simulink model "forward_VAE"  (R2021b)
settings: Solver=FixedStepDiscrete  StartTime=0.0  StopTime=10.0  RelTol=1e-3
PreLoadFcn:
  | CWL=24;
  | CFL=16;
  | CWL_W2=32;
  | CFL_W2=24;
  | CWL_W3=32;
  | CFL_W3=24;
InitFcn:
  | CWL=24;
  | CFL=16;
  | CWL_W2=32;
  | CFL_W2=24;
  | CWL_W3=32;
  | CFL_W3=24;
settings Model: Creator=Kuro  LastModifiedBy=Kuro
settings SolverCC: AlgebraicLoopSolver=TrustRegion
settings OptimizationCC: BlockReduction=off  ConditionallyExecuteInputs=off  DefaultParameterBehavior=Inlined
settings DebuggingCC: AlgebraicLoopMsg=error  SFMachineParentedDataDiag=warning
settings HardwareCC: ProdBitPerPointer=32  ProdBitPerSizeT=32  ProdBitPerPtrDiffT=32  ProdLargestAtomicFloat=None  ProdIntDivRoundTo=Undefined  ProdEndianess=Unspecified  ProdWordSize=32  ProdHWDeviceType=ASIC/FPGA->ASIC/FPGA  TargetBitPerPointer=64  TargetBitPerSizeT=64  TargetBitPerPtrDiffT=64  TargetLongLongMode=on  TargetIntDivRoundTo=Zero  TargetEndianess=LittleEndian  TargetWordSize=64  TargetHWDeviceType=Custom Processor->MATLAB Host Computer  ProdEqTarget=off

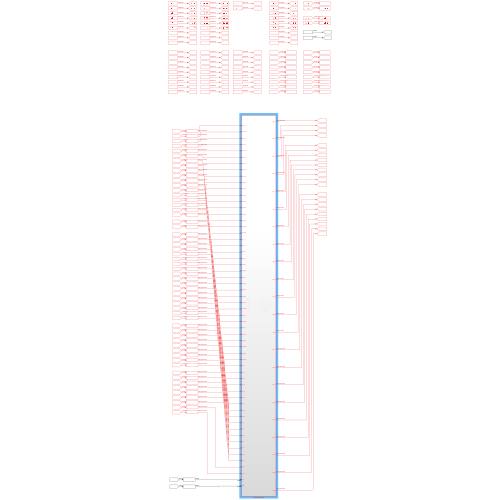
[thumbnail: Simulink's stored preview of the top-level diagram]
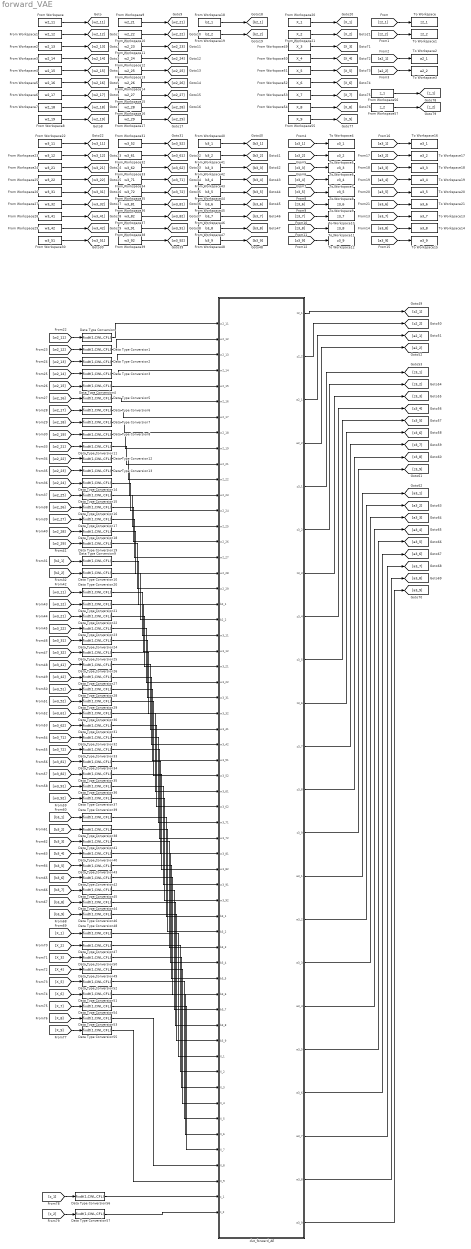
== system forward_VAE ==
  Data Type Conversion{,1..57} (58 alike) : DataTypeConversion  OutDataTypeStr=fixdt(1,CWL,CFL)  SaturateOnIntegerOverflow=on
  From Workspace : FromWorkspace  VariableName=w2_11  SampleTime=1
  From Workspace1 : FromWorkspace  VariableName=w2_12  SampleTime=1
  From Workspace10 : FromWorkspace  VariableName=w2_22  SampleTime=1
  From Workspace11 : FromWorkspace  VariableName=w2_23  SampleTime=1
  From Workspace12 : FromWorkspace  VariableName=w2_24  SampleTime=1
  From Workspace13 : FromWorkspace  VariableName=w2_25  SampleTime=1
  From Workspace14 : FromWorkspace  VariableName=w2_26  SampleTime=1
  From Workspace15 : FromWorkspace  VariableName=w2_27  SampleTime=1
  From Workspace16 : FromWorkspace  VariableName=w2_28  SampleTime=1
  From Workspace17 : FromWorkspace  VariableName=w2_29  SampleTime=1
  From Workspace18 : FromWorkspace  VariableName=b2_1  SampleTime=1
  From Workspace19 : FromWorkspace  VariableName=b2_2  SampleTime=1
  From Workspace2 : FromWorkspace  VariableName=w2_13  SampleTime=1
  From Workspace20 : FromWorkspace  VariableName=X_1  SampleTime=1
  From Workspace21 : FromWorkspace  VariableName=X_2  SampleTime=1
  From Workspace22 : FromWorkspace  VariableName=w3_11  SampleTime=1
  From Workspace23 : FromWorkspace  VariableName=w3_12  SampleTime=1
  From Workspace24 : FromWorkspace  VariableName=w3_21  SampleTime=1
  From Workspace25 : FromWorkspace  VariableName=w3_22  SampleTime=1
  From Workspace26 : FromWorkspace  VariableName=w3_31  SampleTime=1
  From Workspace27 : FromWorkspace  VariableName=w3_32  SampleTime=1
  From Workspace28 : FromWorkspace  VariableName=w3_41  SampleTime=1
  From Workspace29 : FromWorkspace  VariableName=w3_42  SampleTime=1
  From Workspace3 : FromWorkspace  VariableName=w2_14  SampleTime=1
  From Workspace30 : FromWorkspace  VariableName=w3_51  SampleTime=1
  From Workspace31 : FromWorkspace  VariableName=w3_52  SampleTime=1
  From Workspace32 : FromWorkspace  VariableName=w3_61  SampleTime=1
  From Workspace33 : FromWorkspace  VariableName=w3_62  SampleTime=1
  From Workspace34 : FromWorkspace  VariableName=w3_71  SampleTime=1
  From Workspace35 : FromWorkspace  VariableName=w3_72  SampleTime=1
  From Workspace36 : FromWorkspace  VariableName=w3_81  SampleTime=1
  From Workspace37 : FromWorkspace  VariableName=w3_82  SampleTime=1
  From Workspace38 : FromWorkspace  VariableName=w3_91  SampleTime=1
  From Workspace39 : FromWorkspace  VariableName=w3_92  SampleTime=1
  From Workspace4 : FromWorkspace  VariableName=w2_15  SampleTime=1
  From Workspace40 : FromWorkspace  VariableName=b3_1  SampleTime=1
  From Workspace41 : FromWorkspace  VariableName=b3_2  SampleTime=1
  From Workspace42 : FromWorkspace  VariableName=b3_3  SampleTime=1
  From Workspace43 : FromWorkspace  VariableName=b3_4  SampleTime=1
  From Workspace44 : FromWorkspace  VariableName=b3_5  SampleTime=1
  From Workspace45 : FromWorkspace  VariableName=b3_6  SampleTime=1
  From Workspace46 : FromWorkspace  VariableName=b3_7  SampleTime=1
  From Workspace47 : FromWorkspace  VariableName=b3_8  SampleTime=1
  From Workspace48 : FromWorkspace  VariableName=b3_9  SampleTime=1
  From Workspace49 : FromWorkspace  VariableName=X_3  SampleTime=1
  From Workspace5 : FromWorkspace  VariableName=w2_16  SampleTime=1
  From Workspace50 : FromWorkspace  VariableName=X_4  SampleTime=1
  From Workspace51 : FromWorkspace  VariableName=X_5  SampleTime=1
  From Workspace52 : FromWorkspace  VariableName=X_6  SampleTime=1
  From Workspace53 : FromWorkspace  VariableName=X_7  SampleTime=1
  From Workspace54 : FromWorkspace  VariableName=X_8  SampleTime=1
  From Workspace55 : FromWorkspace  VariableName=X_9  SampleTime=1
  From Workspace56 : FromWorkspace  VariableName=z_1  SampleTime=1
  From Workspace57 : FromWorkspace  VariableName=z_2  SampleTime=1
  From Workspace6 : FromWorkspace  VariableName=w2_17  SampleTime=1
  From Workspace7 : FromWorkspace  VariableName=w2_18  SampleTime=1
  From Workspace8 : FromWorkspace  VariableName=w2_19  SampleTime=1
  From Workspace9 : FromWorkspace  VariableName=w2_21  SampleTime=1
  To Workspace : ToWorkspace  VariableName=z2_1  SaveFormat=Timeseries  SampleTime=-1
  To Workspace1 : ToWorkspace  VariableName=z2_2  SaveFormat=Timeseries  SampleTime=-1
  To Workspace10 : ToWorkspace  VariableName=z3_7  SaveFormat=Timeseries  SampleTime=-1
  To Workspace11 : ToWorkspace  VariableName=z3_8  SaveFormat=Timeseries  SampleTime=-1
  To Workspace12 : ToWorkspace  VariableName=z3_9  SaveFormat=Timeseries  SampleTime=-1
  To Workspace13 : ToWorkspace  VariableName=a3_7  SaveFormat=Timeseries  SampleTime=-1
  To Workspace14 : ToWorkspace  VariableName=a3_8  SaveFormat=Timeseries  SampleTime=-1
  To Workspace15 : ToWorkspace  VariableName=a3_9  SaveFormat=Timeseries  SampleTime=-1
  To Workspace16 : ToWorkspace  VariableName=a3_1  SaveFormat=Timeseries  SampleTime=-1
  To Workspace17 : ToWorkspace  VariableName=a3_2  SaveFormat=Timeseries  SampleTime=-1
  To Workspace18 : ToWorkspace  VariableName=a3_3  SaveFormat=Timeseries  SampleTime=-1
  To Workspace19 : ToWorkspace  VariableName=a3_4  SaveFormat=Timeseries  SampleTime=-1
  To Workspace2 : ToWorkspace  VariableName=a2_1  SaveFormat=Timeseries  SampleTime=-1
  To Workspace20 : ToWorkspace  VariableName=a3_5  SaveFormat=Timeseries  SampleTime=-1
  To Workspace21 : ToWorkspace  VariableName=a3_6  SaveFormat=Timeseries  SampleTime=-1
  To Workspace3 : ToWorkspace  VariableName=a2_2  SaveFormat=Timeseries  SampleTime=-1
  To Workspace4 : ToWorkspace  VariableName=z3_1  SaveFormat=Timeseries  SampleTime=-1
  To Workspace5 : ToWorkspace  VariableName=z3_2  SaveFormat=Timeseries  SampleTime=-1
  To Workspace6 : ToWorkspace  VariableName=z3_3  SaveFormat=Timeseries  SampleTime=-1
  To Workspace7 : ToWorkspace  VariableName=z3_4  SaveFormat=Timeseries  SampleTime=-1
  To Workspace8 : ToWorkspace  VariableName=z3_5  SaveFormat=Timeseries  SampleTime=-1
  To Workspace9 : ToWorkspace  VariableName=z3_6  SaveFormat=Timeseries  SampleTime=-1
  dut_forward_AE : Subsystem  TreatAsAtomicUnit=on
  wires:
  From Workspace/1 -> [w2_11]
  From Workspace1/1 -> [w2_12]
  From Workspace3/1 -> [w2_14]
  From Workspace2/1 -> [w2_13]
  From Workspace6/1 -> [w2_17]
  From Workspace5/1 -> [w2_16]
  From Workspace4/1 -> [w2_15]
  From Workspace7/1 -> [w2_18]
  From Workspace8/1 -> [w2_19]
  From Workspace17/1 -> [w2_29]
  From Workspace16/1 -> [w2_28]
  From Workspace13/1 -> [w2_25]
  From Workspace14/1 -> [w2_26]
  From Workspace15/1 -> [w2_27]
  From Workspace11/1 -> [w2_23]
  From Workspace12/1 -> [w2_24]
  From Workspace10/1 -> [w2_22]
  From Workspace9/1 -> [w2_21]
  From Workspace18/1 -> [b2_1]
  From Workspace19/1 -> [b2_2]
  From Workspace30/1 -> [w3_51]
  From Workspace29/1 -> [w3_42]
  From Workspace26/1 -> [w3_31]
  From Workspace27/1 -> [w3_32]
  From Workspace28/1 -> [w3_41]
  From Workspace24/1 -> [w3_21]
  From Workspace25/1 -> [w3_22]
  From Workspace23/1 -> [w3_12]
  From Workspace22/1 -> [w3_11]
  From Workspace31/1 -> [w3_52]
  From Workspace33/1 -> [w3_62]
  From Workspace32/1 -> [w3_61]
  From Workspace36/1 -> [w3_81]
  From Workspace35/1 -> [w3_72]
  From Workspace34/1 -> [w3_71]
  From Workspace37/1 -> [w3_82]
  From Workspace38/1 -> [w3_91]
  From Workspace39/1 -> [w3_92]
  From Workspace40/1 -> [b3_1]
  From Workspace41/1 -> [b3_2]
  From Workspace43/1 -> [b3_4]
  From Workspace42/1 -> [b3_3]
  From Workspace46/1 -> [b3_7]
  From Workspace47/1 -> [b3_8]
  From Workspace45/1 -> [b3_6]
  From Workspace44/1 -> [b3_5]
  From Workspace48/1 -> [b3_9]
  [z2_1] -> To Workspace/1
  [z2_2] -> To Workspace1/1
  [a2_2] -> To Workspace3/1
  [a2_1] -> To Workspace2/1
  [z3_2] -> To Workspace5/1
  [z3_1] -> To Workspace4/1
  [z3_3] -> To Workspace6/1
  [z3_4] -> To Workspace7/1
  [z3_8] -> To Workspace11/1
  [z3_7] -> To Workspace10/1
  [z3_5] -> To Workspace8/1
  [z3_6] -> To Workspace9/1
  [z3_9] -> To Workspace12/1
  [a3_9] -> To Workspace15/1
  [a3_6] -> To Workspace21/1
  [a3_5] -> To Workspace20/1
  [a3_7] -> To Workspace13/1
  [a3_8] -> To Workspace14/1
  [a3_4] -> To Workspace19/1
  [a3_3] -> To Workspace18/1
  [a3_1] -> To Workspace16/1
  [a3_2] -> To Workspace17/1
  [w2_11] -> Data Type Conversion/1
  [w2_12] -> Data Type Conversion1/1
  [w2_14] -> Data Type Conversion3/1
  [w2_13] -> Data Type Conversion2/1
  [w2_17] -> Data Type Conversion6/1
  [w2_18] -> Data Type Conversion7/1
  [w2_16] -> Data Type Conversion5/1
  [w2_15] -> Data Type Conversion4/1
  [w2_19] -> Data Type Conversion8/1
  [b2_1] -> Data Type Conversion9/1
  [w2_29] -> Data Type Conversion19/1
  [w2_25] -> Data Type Conversion15/1
  [w2_26] -> Data Type Conversion16/1
  [w2_28] -> Data Type Conversion18/1
  [w2_27] -> Data Type Conversion17/1
  [w2_23] -> Data Type Conversion13/1
  [w2_24] -> Data Type Conversion14/1
  [w2_22] -> Data Type Conversion12/1
  [w2_21] -> Data Type Conversion11/1
  [b2_2] -> Data Type Conversion10/1
  [w3_12] -> Data Type Conversion21/1
  [w3_11] -> Data Type Conversion20/1
  [w3_21] -> Data Type Conversion22/1
  [w3_22] -> Data Type Conversion23/1
  [w3_42] -> Data Type Conversion27/1
  [w3_41] -> Data Type Conversion26/1
  [w3_31] -> Data Type Conversion24/1
  [w3_32] -> Data Type Conversion25/1
  [w3_72] -> Data Type Conversion33/1
  [w3_71] -> Data Type Conversion32/1
  [w3_81] -> Data Type Conversion34/1
  [w3_62] -> Data Type Conversion31/1
  [w3_61] -> Data Type Conversion30/1
  [w3_51] -> Data Type Conversion28/1
  [w3_52] -> Data Type Conversion29/1
  [w3_82] -> Data Type Conversion35/1
  [w3_92] -> Data Type Conversion37/1
  [w3_91] -> Data Type Conversion36/1
  [b3_2] -> Data Type Conversion38/1
  [b3_1] -> Data Type Conversion39/1
  [b3_3] -> Data Type Conversion41/1
  [b3_4] -> Data Type Conversion40/1
  [b3_8] -> Data Type Conversion44/1
  [b3_7] -> Data Type Conversion45/1
  [b3_5] -> Data Type Conversion43/1
  [b3_6] -> Data Type Conversion42/1
  [b3_9] -> Data Type Conversion46/1
  [X_1] -> Data Type Conversion48/1
  [X_2] -> Data Type Conversion47/1
  From Workspace55/1 -> [X_9]
  From Workspace51/1 -> [X_5]
  From Workspace52/1 -> [X_6]
  From Workspace54/1 -> [X_8]
  From Workspace53/1 -> [X_7]
  From Workspace49/1 -> [X_3]
  From Workspace50/1 -> [X_4]
  From Workspace21/1 -> [X_2]
  From Workspace20/1 -> [X_1]
  [X_4] -> Data Type Conversion49/1
  [X_3] -> Data Type Conversion50/1
  [X_7] -> Data Type Conversion54/1
  [X_8] -> Data Type Conversion53/1
  [X_6] -> Data Type Conversion51/1
  [X_5] -> Data Type Conversion52/1
  [X_9] -> Data Type Conversion55/1
  Data Type Conversion/1 -> dut_forward_AE/1(w2_11)
  Data Type Conversion1/1 -> dut_forward_AE/2(w2_12)
  Data Type Conversion2/1 -> dut_forward_AE/3(w2_13)
  Data Type Conversion3/1 -> dut_forward_AE/4(w2_14)
  Data Type Conversion4/1 -> dut_forward_AE/5(w2_15)
  Data Type Conversion5/1 -> dut_forward_AE/6(w2_16)
  Data Type Conversion6/1 -> dut_forward_AE/7(w2_17)
  Data Type Conversion7/1 -> dut_forward_AE/8(w2_18)
  Data Type Conversion8/1 -> dut_forward_AE/9(w2_19)
  Data Type Conversion11/1 -> dut_forward_AE/10(w2_21)
  Data Type Conversion12/1 -> dut_forward_AE/11(w2_22)
  Data Type Conversion13/1 -> dut_forward_AE/12(w2_23)
  Data Type Conversion14/1 -> dut_forward_AE/13(w2_24)
  Data Type Conversion15/1 -> dut_forward_AE/14(w2_25)
  Data Type Conversion16/1 -> dut_forward_AE/15(w2_26)
  Data Type Conversion17/1 -> dut_forward_AE/16(w2_27)
  Data Type Conversion18/1 -> dut_forward_AE/17(w2_28)
  Data Type Conversion19/1 -> dut_forward_AE/18(w2_29)
  Data Type Conversion9/1 -> dut_forward_AE/19(b2_1)
  Data Type Conversion10/1 -> dut_forward_AE/20(b2_2)
  Data Type Conversion20/1 -> dut_forward_AE/21(w3_11)
  Data Type Conversion21/1 -> dut_forward_AE/22(w3_12)
  Data Type Conversion22/1 -> dut_forward_AE/23(w3_21)
  Data Type Conversion23/1 -> dut_forward_AE/24(w3_22)
  Data Type Conversion24/1 -> dut_forward_AE/25(w3_31)
  Data Type Conversion25/1 -> dut_forward_AE/26(w3_32)
  Data Type Conversion26/1 -> dut_forward_AE/27(w3_41)
  Data Type Conversion27/1 -> dut_forward_AE/28(w3_42)
  Data Type Conversion28/1 -> dut_forward_AE/29(w3_51)
  Data Type Conversion29/1 -> dut_forward_AE/30(w3_52)
  Data Type Conversion30/1 -> dut_forward_AE/31(w3_61)
  Data Type Conversion31/1 -> dut_forward_AE/32(w3_62)
  Data Type Conversion32/1 -> dut_forward_AE/33(w3_71)
  Data Type Conversion33/1 -> dut_forward_AE/34(w3_72)
  Data Type Conversion34/1 -> dut_forward_AE/35(w3_81)
  Data Type Conversion35/1 -> dut_forward_AE/36(w3_82)
  Data Type Conversion36/1 -> dut_forward_AE/37(w3_91)
  Data Type Conversion37/1 -> dut_forward_AE/38(w3_92)
  Data Type Conversion39/1 -> dut_forward_AE/39(b3_1)
  Data Type Conversion38/1 -> dut_forward_AE/40(b3_2)
  Data Type Conversion41/1 -> dut_forward_AE/41(b3_3)
  Data Type Conversion40/1 -> dut_forward_AE/42(b3_4)
  Data Type Conversion43/1 -> dut_forward_AE/43(b3_5)
  Data Type Conversion42/1 -> dut_forward_AE/44(b3_6)
  Data Type Conversion45/1 -> dut_forward_AE/45(b3_7)
  Data Type Conversion44/1 -> dut_forward_AE/46(b3_8)
  Data Type Conversion46/1 -> dut_forward_AE/47(b3_9)
  Data Type Conversion48/1 -> dut_forward_AE/48(X_1)
  Data Type Conversion47/1 -> dut_forward_AE/49(X_2)
  Data Type Conversion50/1 -> dut_forward_AE/50(X_3)
  Data Type Conversion49/1 -> dut_forward_AE/51(X_4)
  Data Type Conversion52/1 -> dut_forward_AE/52(X_5)
  Data Type Conversion51/1 -> dut_forward_AE/53(X_6)
  Data Type Conversion54/1 -> dut_forward_AE/54(X_7)
  Data Type Conversion53/1 -> dut_forward_AE/55(X_8)
  Data Type Conversion55/1 -> dut_forward_AE/56(X_9)
  dut_forward_AE/1(z2_1) -> [z2_1]
  dut_forward_AE/2(z2_2) -> [z2_2]
  dut_forward_AE/3(a2_1) -> [a2_1]
  dut_forward_AE/4(a2_2) -> [a2_2]
  dut_forward_AE/5(z3_1) -> [z3_1]
  dut_forward_AE/6(z3_2) -> [z3_2]
  dut_forward_AE/7(z3_3) -> [z3_3]
  dut_forward_AE/8(z3_4) -> [z3_4]
  dut_forward_AE/9(z3_5) -> [z3_5]
  dut_forward_AE/10(z3_6) -> [z3_6]
  dut_forward_AE/11(z3_7) -> [z3_7]
  dut_forward_AE/12(z3_8) -> [z3_8]
  dut_forward_AE/13(z3_9) -> [z3_9]
  dut_forward_AE/14(a3_1) -> [a3_1]
  dut_forward_AE/15(a3_2) -> [a3_2]
  dut_forward_AE/16(a3_3) -> [a3_3]
  dut_forward_AE/17(a3_4) -> [a3_4]
  dut_forward_AE/18(a3_5) -> [a3_5]
  dut_forward_AE/19(a3_6) -> [a3_6]
  dut_forward_AE/20(a3_7) -> [a3_7]
  dut_forward_AE/21(a3_8) -> [a3_8]
  dut_forward_AE/22(a3_9) -> [a3_9]
  From Workspace56/1 -> [z_1]
  From Workspace57/1 -> [z_2]
  [z_1] -> Data Type Conversion56/1
  [z_2] -> Data Type Conversion57/1
  Data Type Conversion56/1 -> dut_forward_AE/57(z_1)
  Data Type Conversion57/1 -> dut_forward_AE/58(z_2)

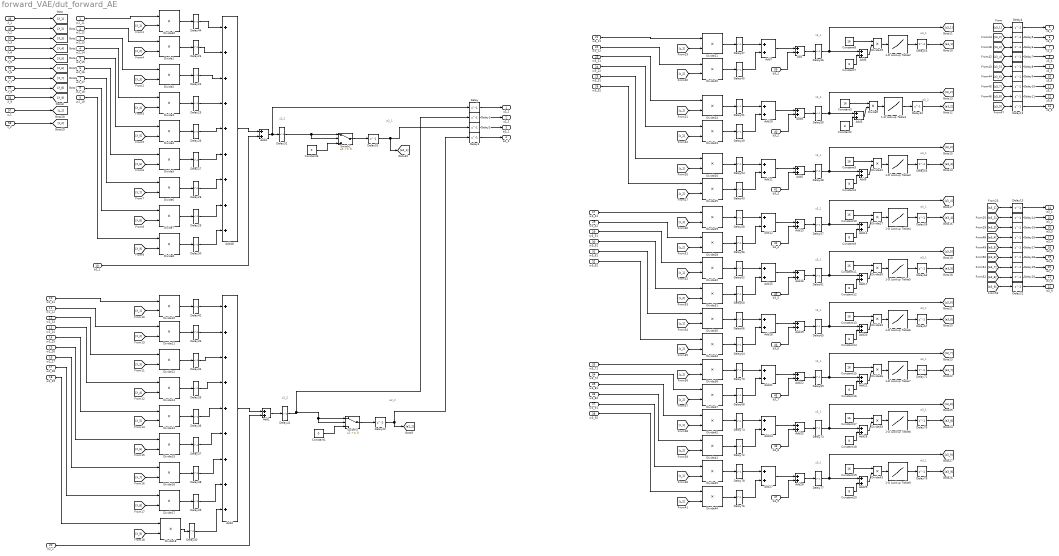
== system forward_VAE/dut_forward_AE ==
  note: a2_1
  note: z2_1
  note: a2_2
  note: z2_2
  note: z3_1
  note: a3_1
  note: z3_2
  note: a3_2
  note: z3_1
  note: a3_1
  note: z3_1
  note: a3_1
  note: z3_1
  note: a3_1
  note: z3_1
  note: a3_1
  note: z3_1
  note: a3_1
  note: z3_1
  note: a3_1
  note: z3_1
  note: a3_1
  w2_11 : Inport
  w2_12 : Inport  Port=2
  w2_13 : Inport  Port=3
  w2_14 : Inport  Port=4
  w2_15 : Inport  Port=5
  w2_16 : Inport  Port=6
  w2_17 : Inport  Port=7
  w2_18 : Inport  Port=8
  w2_19 : Inport  Port=9
  w2_21 : Inport  Port=10
  w2_22 : Inport  Port=11
  w2_23 : Inport  Port=12
  w2_24 : Inport  Port=13
  w2_25 : Inport  Port=14
  w2_26 : Inport  Port=15
  w2_27 : Inport  Port=16
  w2_28 : Inport  Port=17
  w2_29 : Inport  Port=18
  b2_1 : Inport  Port=19
  b2_2 : Inport  Port=20
  w3_11 : Inport  Port=21
  w3_12 : Inport  Port=22
  w3_21 : Inport  Port=23
  w3_22 : Inport  Port=24
  w3_31 : Inport  Port=25
  w3_32 : Inport  Port=26
  w3_41 : Inport  Port=27
  w3_42 : Inport  Port=28
  w3_51 : Inport  Port=29
  w3_52 : Inport  Port=30
  w3_61 : Inport  Port=31
  w3_62 : Inport  Port=32
  w3_71 : Inport  Port=33
  w3_72 : Inport  Port=34
  w3_81 : Inport  Port=35
  w3_82 : Inport  Port=36
  w3_91 : Inport  Port=37
  w3_92 : Inport  Port=38
  b3_1 : Inport  Port=39
  b3_2 : Inport  Port=40
  b3_3 : Inport  Port=41
  b3_4 : Inport  Port=42
  b3_5 : Inport  Port=43
  b3_6 : Inport  Port=44
  b3_7 : Inport  Port=45
  b3_8 : Inport  Port=46
  b3_9 : Inport  Port=47
  X_1 : Inport  Port=48
  X_2 : Inport  Port=49
  X_3 : Inport  Port=50
  X_4 : Inport  Port=51
  X_5 : Inport  Port=52
  X_6 : Inport  Port=53
  X_7 : Inport  Port=54
  X_8 : Inport  Port=55
  X_9 : Inport  Port=56
  z_1 : Inport  Port=57
  z_2 : Inport  Port=58
  1-D Lookup Table{1..9} (9 alike) : Lookup_n-D  NumberOfTableDimensions=1  LookupTableObject=''  BreakpointsForDimension1=[0:255]  BreakpointsForDimension1FirstPoint=10  BreakpointsForDimension2FirstPoint=10  BreakpointsForDimension1Spacing=12  BreakpointsForDimension2Spacing=12  IndexSearchMethod=Evenly spaced points  Table=1./(1+exp(-1*[-8:2^(-4):8-2^(-4)]))  InterpMethod=Flat  DiagnosticForOutOfRangeInput=Error  OutDataTypeStr=fixdt(1,CWL,CFL)  RndMeth=Simplest  SaturateOnIntegerOverflow=on  InputSameDT=on
  Add{,5,8,13,16,19,22,25,28} (9 alike) : Sum  AccumDataTypeStr=fixdt(1,CWL_W3,CFL_W3)  OutDataTypeStr=fixdt(1,8,4)  RndMeth=Round  SaturateOnIntegerOverflow=on
  Add1 : Sum  AccumDataTypeStr=fixdt(1,CWL_W2,CFL_W2)  OutDataTypeStr=fixdt(1,CWL,CFL)  RndMeth=Round  SaturateOnIntegerOverflow=on
  Add{7,10..12,15,18,21,24,27} (9 alike) : Sum  AccumDataTypeStr=fixdt(1,CWL_W3,CFL_W3)  OutDataTypeStr=fixdt(1,CWL_W3,CFL_W3)  RndMeth=Round  SaturateOnIntegerOverflow=on
  Add{3,6,9,14,17,20,23,26,29} (9 alike) : Sum  AccumDataTypeStr=fixdt(1,16,8)  OutDataTypeStr=fixdt(0,8,4)  RndMeth=Round  SaturateOnIntegerOverflow=on
  Add2 : Sum  Inputs=+++++++++  AccumDataTypeStr=fixdt(1,CWL_W2,CFL_W2)  OutDataTypeStr=fixdt(1,CWL_W2,CFL_W2)  RndMeth=Round  SaturateOnIntegerOverflow=on
  Add4 : Sum  AccumDataTypeStr=fixdt(1,CWL_W2,CFL_W2)  OutDataTypeStr=fixdt(1,CWL,CFL)  RndMeth=Round  SaturateOnIntegerOverflow=on
  Add48 : Sum  Inputs=+++++++++  AccumDataTypeStr=fixdt(1,CWL_W2,CFL_W2)  OutDataTypeStr=fixdt(1,CWL_W2,CFL_W2)  RndMeth=Round  SaturateOnIntegerOverflow=on
  Constant1 : Constant  Value=0  OutDataTypeStr=fixdt(1,CWL,CFL)  SampleTime=-1
  Constant{3,5,8,10..11,13,15,17,19} (9 alike) : Constant  Value=16  OutDataTypeStr=fixdt(0,8,0)  SampleTime=1
  Constant{2,4,7,9,12,14,16,18,20} (9 alike) : Constant  Value=8  OutDataTypeStr=fixdt(1,16,8)  SampleTime=1
  Constant6 : Constant  Value=0  OutDataTypeStr=fixdt(1,CWL,CFL)  SampleTime=-1
  Delay{,1..79} (80 alike) : Delay  DelayLength=1  InitialCondition=0
  Divide{1..8,10..18,40} (18 alike) : Product  Inputs=**  OutDataTypeStr=fixdt(1,CWL_W2,CFL_W2)  RndMeth=Round  SaturateOnIntegerOverflow=on
  Divide{9,19,22,27,30,33,36,39,43} (9 alike) : Product  Inputs=**  OutDataTypeStr=fixdt(0,8,0)  RndMeth=Round  SaturateOnIntegerOverflow=on
  Divide{20..21,23..26,28..29,31..32,34..35,37..38,41..42,44..45} (18 alike) : Product  Inputs=**  OutDataTypeStr=fixdt(1,CWL_W3,CFL_W3)  RndMeth=Round  SaturateOnIntegerOverflow=on
  Switch2 : Switch
  Switch3 : Switch
  z2_1 : Outport
  z2_2 : Outport  Port=2
  a2_1 : Outport  Port=3
  a2_2 : Outport  Port=4
  z3_1 : Outport  Port=5
  z3_2 : Outport  Port=6
  z3_3 : Outport  Port=7
  z3_4 : Outport  Port=8
  z3_5 : Outport  Port=9
  z3_6 : Outport  Port=10
  z3_7 : Outport  Port=11
  z3_8 : Outport  Port=12
  z3_9 : Outport  Port=13
  a3_1 : Outport  Port=14
  a3_2 : Outport  Port=15
  a3_3 : Outport  Port=16
  a3_4 : Outport  Port=17
  a3_5 : Outport  Port=18
  a3_6 : Outport  Port=19
  a3_7 : Outport  Port=20
  a3_8 : Outport  Port=21
  a3_9 : Outport  Port=22
  wires:
  Delay13/1 -> a3_1/1
  X_3/1 -> [X_3]
  Delay9/1 -> z3_6/1
  X_1/1 -> [X_1]
  Delay4/1 -> z3_1/1
  Delay19/1 -> a3_7/1
  Delay12/1 -> z3_9/1
  X_5/1 -> [X_5]
  Delay17/1 -> a3_5/1
  Delay16/1 -> a3_4/1
  Delay6/1 -> z3_3/1
  Delay/1 -> z2_1/1
  Delay7/1 -> z3_4/1
  Delay2/1 -> a2_1/1
  Delay18/1 -> a3_6/1
  Delay3/1 -> a2_2/1
  Delay20/1 -> a3_8/1
  Delay5/1 -> z3_2/1
  Delay14/1 -> a3_2/1
  Delay10/1 -> z3_7/1
  Delay11/1 -> z3_8/1
  Delay1/1 -> z2_2/1
  Delay15/1 -> a3_3/1
  X_2/1 -> [X_2]
  X_6/1 -> [X_6]
  X_4/1 -> [X_4]
  X_7/1 -> [X_7]
  X_9/1 -> [X_9]
  X_8/1 -> [X_8]
  Delay21/1 -> a3_9/1
  Delay8/1 -> z3_5/1
  Divide1/1 -> Delay23/1
  [X_2] -> Divide1/2
  w2_12/1 -> Divide1/1
  Delay23/1 -> Add48/2
  [X_1] -> Divide40/2
  w2_11/1 -> Divide40/1
  Add48/1 -> Add4/1
  Delay44/1 -> Add48/1
  Add4/1 -> Delay/1, Delay31/1
  Divide40/1 -> Delay44/1
  Delay24/1 -> Add48/3
  [X_3] -> Divide2/2
  Divide2/1 -> Delay24/1
  Divide3/1 -> Delay25/1
  [X_4] -> Divide3/2
  Delay25/1 -> Add48/4
  Delay26/1 -> Add48/5
  [X_5] -> Divide4/2
  Divide4/1 -> Delay26/1
  Divide5/1 -> Delay27/1
  [X_6] -> Divide5/2
  Delay27/1 -> Add48/6
  Delay28/1 -> Add48/7
  [X_7] -> Divide6/2
  Divide6/1 -> Delay28/1
  Divide7/1 -> Delay29/1
  [X_8] -> Divide7/2
  Delay29/1 -> Add48/8
  Delay30/1 -> Add48/9
  [X_9] -> Divide8/2
  Divide8/1 -> Delay30/1
  w2_13/1 -> Divide2/1
  w2_14/1 -> Divide3/1
  w2_15/1 -> Divide4/1
  w2_16/1 -> Divide5/1
  w2_17/1 -> Divide6/1
  w2_18/1 -> Divide7/1
  w2_19/1 -> Divide8/1
  w2_29/1 -> Divide18/1
  w2_28/1 -> Divide17/1
  w2_27/1 -> Divide16/1
  w2_26/1 -> Divide15/1
  w2_25/1 -> Divide14/1
  w2_24/1 -> Divide13/1
  w2_23/1 -> Divide12/1
  Divide18/1 -> Delay40/1
  [X_9] -> Divide18/2
  Delay40/1 -> Add2/9
  Delay39/1 -> Add2/8
  [X_8] -> Divide17/2
  Divide17/1 -> Delay39/1
  Divide16/1 -> Delay38/1
  [X_7] -> Divide16/2
  Delay38/1 -> Add2/7
  Delay37/1 -> Add2/6
  [X_6] -> Divide15/2
  Divide15/1 -> Delay37/1
  Divide14/1 -> Delay36/1
  [X_5] -> Divide14/2
  Delay36/1 -> Add2/5
  Delay35/1 -> Add2/4
  [X_4] -> Divide13/2
  Divide13/1 -> Delay35/1
  Divide12/1 -> Delay34/1
  [X_3] -> Divide12/2
  Delay34/1 -> Add2/3
  Divide10/1 -> Delay42/1
  Add1/1 -> Delay41/1
  Delay42/1 -> Add2/1
  Add2/1 -> Add1/1
  [X_1] -> Divide10/2
  Delay33/1 -> Add2/2
  w2_22/1 -> Divide11/1
  [X_2] -> Divide11/2
  Divide11/1 -> Delay33/1
  w2_21/1 -> Divide10/1
  b2_2/1 -> Add1/2
  b2_1/1 -> Add4/2
  Divide21/1 -> Delay47/1
  Divide20/1 -> Delay45/1
  [z_2] -> Divide20/2
  Delay47/1 -> Add7/1
  Add7/1 -> Add/1
  Delay45/1 -> Add7/2
  Add/1 -> Delay46/1
  [z_1] -> Divide21/2
  Add8/1 -> Delay50/1
  Delay49/1 -> Add10/2
  Delay51/1 -> Add10/1
  Divide24/1 -> Delay51/1
  [z_1] -> Divide24/2
  [z_2] -> Divide23/2
  Add10/1 -> Add8/1
  Divide23/1 -> Delay49/1
  w3_11/1 -> Divide21/1
  w3_12/1 -> Divide20/1
  w3_21/1 -> Divide24/1
  w3_22/1 -> Divide23/1
  b3_1/1 -> Add/2
  b3_2/1 -> Add8/2
  Constant6/1 -> Switch2/3
  Switch2/1 -> Delay52/1
  Delay31/1 -> Switch2/1, Switch2/2
  1-D Lookup Table2/1 -> Delay53/1
  Constant7/1 -> Add6/2
  Divide19/1 -> 1-D Lookup Table2/1
  Delay46/1 -> Add6/1, [z3_1]
  Add6/1 -> Divide19/2
  Delay52/1 -> [a2_1], Delay2/1
  Constant8/1 -> Divide19/1
  Delay41/1 -> Switch3/2, Switch3/1, Delay1/1
  Switch3/1 -> Delay22/1
  Constant1/1 -> Switch3/3
  Delay22/1 -> Delay3/1, [a2_2]
  Constant3/1 -> Divide9/1
  Add3/1 -> Divide9/2
  Divide9/1 -> 1-D Lookup Table1/1
  Constant2/1 -> Add3/2
  1-D Lookup Table1/1 -> Delay32/1
  Delay53/1 -> [a3_1]
  Delay32/1 -> [a3_2]
  Delay50/1 -> [z3_2], Add3/1
  [z3_1] -> Delay4/1
  [a3_1] -> Delay13/1
  [z3_2] -> Delay5/1
  [a3_2] -> Delay14/1
  Delay55/1 -> [a3_3]
  Constant5/1 -> Divide22/1
  Add9/1 -> Divide22/2
  Delay48/1 -> [z3_3], Add9/1
  Divide22/1 -> 1-D Lookup Table3/1
  Constant4/1 -> Add9/2
  1-D Lookup Table3/1 -> Delay55/1
  [z_1] -> Divide26/2
  Add5/1 -> Delay48/1
  Delay43/1 -> Add11/2
  Add11/1 -> Add5/1
  Delay54/1 -> Add11/1
  [z_2] -> Divide25/2
  Divide25/1 -> Delay43/1
  Divide26/1 -> Delay54/1
  w3_31/1 -> Divide26/1
  w3_32/1 -> Divide25/1
  [z3_3] -> Delay6/1
  [a3_3] -> Delay15/1
  Divide29/1 -> Delay58/1
  Divide28/1 -> Delay56/1
  [z_2] -> Divide28/2
  Delay58/1 -> Add12/1
  Add12/1 -> Add13/1
  Delay56/1 -> Add12/2
  Add13/1 -> Delay57/1
  [z_1] -> Divide29/2
  1-D Lookup Table4/1 -> Delay59/1
  Constant9/1 -> Add14/2
  Divide27/1 -> 1-D Lookup Table4/1
  Delay57/1 -> Add14/1, [z3_4]
  Add14/1 -> Divide27/2
  Constant10/1 -> Divide27/1
  Delay59/1 -> [a3_4]
  Delay63/1 -> [a3_5]
  Constant11/1 -> Divide30/1
  Add17/1 -> Divide30/2
  Delay61/1 -> [z3_5], Add17/1
  Divide30/1 -> 1-D Lookup Table5/1
  Constant12/1 -> Add17/2
  1-D Lookup Table5/1 -> Delay63/1
  [z_1] -> Divide32/2
  Add16/1 -> Delay61/1
  Delay60/1 -> Add15/2
  Add15/1 -> Add16/1
  Delay62/1 -> Add15/1
  [z_2] -> Divide31/2
  Divide31/1 -> Delay60/1
  Divide32/1 -> Delay62/1
  Divide35/1 -> Delay66/1
  Divide34/1 -> Delay64/1
  [z_2] -> Divide34/2
  Delay66/1 -> Add18/1
  Add18/1 -> Add19/1
  Delay64/1 -> Add18/2
  Add19/1 -> Delay65/1
  [z_1] -> Divide35/2
  1-D Lookup Table6/1 -> Delay67/1
  Constant14/1 -> Add20/2
  Divide33/1 -> 1-D Lookup Table6/1
  Delay65/1 -> Add20/1, [z3_6]
  Add20/1 -> Divide33/2
  Constant13/1 -> Divide33/1
  Delay67/1 -> [a3_6]
  Delay71/1 -> [a3_7]
  Constant15/1 -> Divide36/1
  Add23/1 -> Divide36/2
  Delay69/1 -> [z3_7], Add23/1
  Divide36/1 -> 1-D Lookup Table7/1
  Constant16/1 -> Add23/2
  1-D Lookup Table7/1 -> Delay71/1
  [z_1] -> Divide38/2
  Add22/1 -> Delay69/1
  Delay68/1 -> Add21/2
  Add21/1 -> Add22/1
  Delay70/1 -> Add21/1
  [z_2] -> Divide37/2
  Divide37/1 -> Delay68/1
  Divide38/1 -> Delay70/1
  Divide42/1 -> Delay74/1
  Divide41/1 -> Delay72/1
  [z_2] -> Divide41/2
  Delay74/1 -> Add24/1
  Add24/1 -> Add25/1
  Delay72/1 -> Add24/2
  Add25/1 -> Delay73/1
  [z_1] -> Divide42/2
  1-D Lookup Table8/1 -> Delay75/1
  Constant18/1 -> Add26/2
  Divide39/1 -> 1-D Lookup Table8/1
  Delay73/1 -> Add26/1, [z3_8]
  Add26/1 -> Divide39/2
  Constant17/1 -> Divide39/1
  Delay75/1 -> [a3_8]
  Delay79/1 -> [a3_9]
  Constant19/1 -> Divide43/1
  Add29/1 -> Divide43/2
  Delay77/1 -> [z3_9], Add29/1
  Divide43/1 -> 1-D Lookup Table9/1
  Constant20/1 -> Add29/2
  1-D Lookup Table9/1 -> Delay79/1
  [z_1] -> Divide45/2
  Add28/1 -> Delay77/1
  Delay76/1 -> Add27/2
  Add27/1 -> Add28/1
  Delay78/1 -> Add27/1
  [z_2] -> Divide44/2
  Divide44/1 -> Delay76/1
  Divide45/1 -> Delay78/1
  [z3_4] -> Delay7/1
  [z3_5] -> Delay8/1
  [z3_6] -> Delay9/1
  [z3_7] -> Delay10/1
  [z3_8] -> Delay11/1
  [z3_9] -> Delay12/1
  [a3_4] -> Delay16/1
  [a3_5] -> Delay17/1
  [a3_6] -> Delay18/1
  [a3_7] -> Delay19/1
  [a3_8] -> Delay20/1
  [a3_9] -> Delay21/1
  b3_3/1 -> Add5/2
  b3_4/1 -> Add13/2
  b3_5/1 -> Add16/2
  b3_6/1 -> Add19/2
  b3_7/1 -> Add22/2
  b3_8/1 -> Add25/2
  b3_9/1 -> Add28/2
  w3_41/1 -> Divide29/1
  w3_42/1 -> Divide28/1
  w3_51/1 -> Divide32/1
  w3_52/1 -> Divide31/1
  w3_61/1 -> Divide35/1
  w3_62/1 -> Divide34/1
  w3_92/1 -> Divide44/1
  w3_91/1 -> Divide45/1
  w3_82/1 -> Divide41/1
  w3_81/1 -> Divide42/1
  w3_72/1 -> Divide37/1
  w3_71/1 -> Divide38/1
  z_1/1 -> [z_1]
  z_2/1 -> [z_2]
